simulink model "prac3s2022a"  (R2022a)
settings: Solver=ode23t  StartTime=0.0  StopTime=Tmdl  MaxStep=1e-4  RelTol=1e-3
undefined symbols (not defined in the file): Cp, Fext, Kc, Kd, Kf, Ku, Kv, Kx, m, Tu
settings Model: Creator=hdu  LastModifiedBy=86156

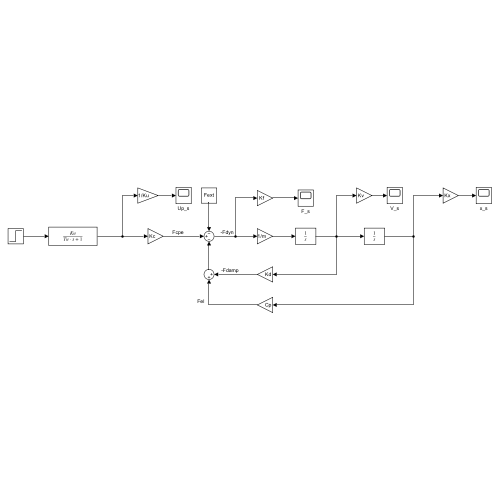
[thumbnail: Simulink's stored preview of the top-level diagram]
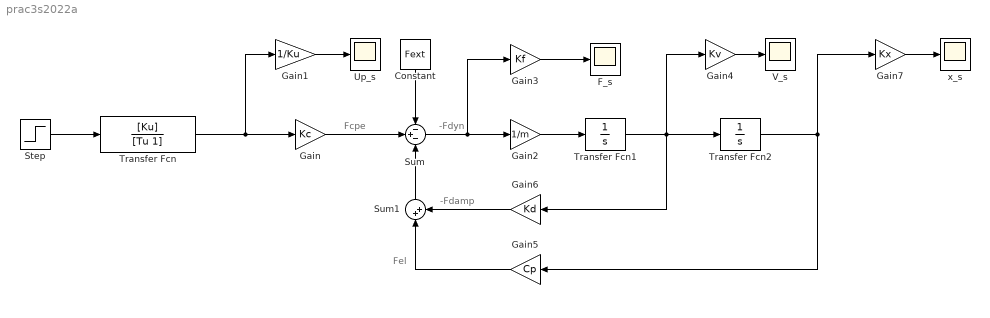
== system prac3s2022a ==
  note: -Fdyn
  note: Fcpe
  note: -Fdamp
  note: Fel
  Constant : Constant  Value=Fext
  F_s : Scope
  Gain : Gain  Gain=Kc
  Gain1 : Gain  Gain=1/Ku
  Gain2 : Gain  Gain=1/m
  Gain3 : Gain  Gain=Kf
  Gain4 : Gain  Gain=Kv
  Gain5 : Gain  Gain=Cp
  Gain6 : Gain  Gain=Kd
  Gain7 : Gain  Gain=Kx
  Step : Step  Time=0  After=u  SampleTime=0
  Sum : Sum  Inputs=-+-
  Sum1 : Sum  Inputs=|++
  Transfer Fcn : TransferFcn  Numerator=[Ku]  Denominator=[Tu 1]
  Transfer Fcn1 : TransferFcn  Denominator=[1 0]
  Transfer Fcn2 : TransferFcn  Denominator=[1 0]
  Up_s : Scope
  V_s : Scope
  x_s : Scope
  wires:
  Transfer Fcn/1 -> Gain1/1, Gain/1
  Step/1 -> Transfer Fcn/1
  Gain/1 -> Sum/2
  Sum/1 -> Gain3/1, Gain2/1
  Gain2/1 -> Transfer Fcn1/1
  Transfer Fcn1/1 -> Transfer Fcn2/1, Gain6/1, Gain4/1
  Sum1/1 -> Sum/3
  Gain6/1 -> Sum1/2
  Gain5/1 -> Sum1/1
  Transfer Fcn2/1 -> Gain7/1, Gain5/1
  Gain1/1 -> Up_s/1
  Gain3/1 -> F_s/1
  Gain4/1 -> V_s/1
  Gain7/1 -> x_s/1
  Constant/1 -> Sum/1
